simulink library "VehicleController_cl"  (R2020a)
settings: Solver=VariableStepAuto  StartTime=0.0  StopTime=10.0  RelTol=1e-3
undefined symbols (not defined in the file): TRAN
libraries: Infrastructure_CL x1, PowertrainController_ul x1, Traffic_2_UL x1, VelocityController_CL x1
settings Model: Creator=John Jr  LastModifiedBy=John Jr

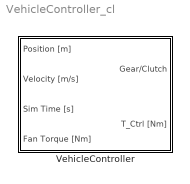
== system VehicleController_cl ==
  VehicleController : Subsystem

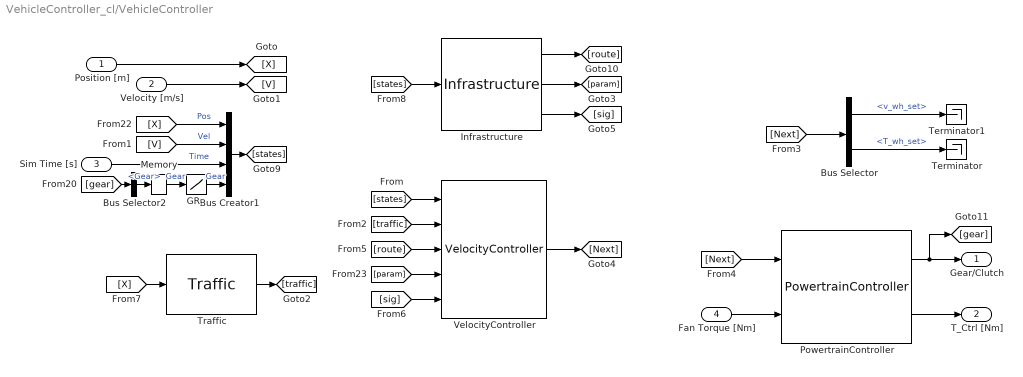
== system VehicleController_cl/VehicleController ==
  Position [m] : Inport
  Velocity [m/s] : Inport  Port=2
  Sim Time [s] : Inport  Port=3
  Fan Torque [Nm] : Inport  Port=4
  Bus Creator1 : BusCreator  Inputs=4
  Bus Selector : BusSelector  OutputSignals=v_wh_set,T_wh_set
  Bus Selector2 : BusSelector  OutputSignals=Gear
  GR : Lookup_n-D  NumberOfTableDimensions=1  BreakpointsForDimension1=[1:TRAN.numGears]  Table=TRAN.gears  ExtrapMethod=Clip  UseLastTableValue=on  InternalRulePriority=Speed  RndMeth=Simplest  InputSameDT=on
  Infrastructure : Infrastructure_CL/Infrastructure  SystemSampleTime=-1  Latency=0  AutoFrameSizeCalculation=off
  Memory : Memory  InitialCondition=11
  PowertrainController : PowertrainController_ul/PowertrainController  SystemSampleTime=-1  Latency=0  AutoFrameSizeCalculation=off
  Terminator : Terminator
  Terminator1 : Terminator
  Traffic : Traffic_2_UL/Traffic  SystemSampleTime=-1  Latency=0  AutoFrameSizeCalculation=off
  VelocityController : VelocityController_CL/VelocityController  SystemSampleTime=-1  Latency=0  AutoFrameSizeCalculation=off
  Gear/Clutch : Outport  VectorParamsAs1DForOutWhenUnconnected=off
  T_Ctrl [Nm] : Outport  Port=2  VectorParamsAs1DForOutWhenUnconnected=off
  wires:
  Bus Selector2/1 -> Memory/1  "<Gear>"
  Velocity [m/s]/1 -> [V]
  Sim Time [s]/1 -> Bus Creator1/3  "Time"
  [traffic] -> VelocityController/2
  [route] -> VelocityController/3
  [gear] -> Bus Selector2/1
  [V] -> Bus Creator1/2  "Vel"
  Position [m]/1 -> [X]
  Bus Creator1/1 -> [states]
  VelocityController/1 -> [Next]
  [states] -> VelocityController/1
  Bus Selector/2 -> Terminator/1  "<T_wh_set>"
  [X] -> Bus Creator1/1  "Pos"
  [Next] -> Bus Selector/1
  Bus Selector/1 -> Terminator1/1  "<v_wh_set>"
  [Next] -> PowertrainController/1
  Fan Torque [Nm]/1 -> PowertrainController/2
  PowertrainController/1 -> Gear/Clutch/1, [gear]
  PowertrainController/2 -> T_Ctrl [Nm]/1
  Infrastructure/1 -> [route]
  [param] -> VelocityController/4
  Infrastructure/2 -> [param]
  Infrastructure/3 -> [sig]
  [sig] -> VelocityController/5
  Memory/1 -> GR/1  "Gear"
  GR/1 -> Bus Creator1/4  "Gear"
  [X] -> Traffic/1
  Traffic/1 -> [traffic]
  [states] -> Infrastructure/1
